simulink model "ProcessSerial"  (R2020a)
settings: Solver=FixedStepAuto  StartTime=0.0  StopTime=10.0  FixedStep=1e-3  RelTol=1e-3  EnableMultiTasking=on
libraries: frdmk64flib x5, simulink x3, etargetslib x1
settings Model: ExtModeTrigDuration=5  Creator=WinnieTrandinh  LastModifiedBy=WinnieTrandinh
settings OptimizationCC: EnhancedBackFolding=on  PassReuseOutputArgsAs=Individual arguments  ZeroExternalMemoryAtStartup=off  ZeroInternalMemoryAtStartup=off  MaxStackSize=64  OptimizeBlockOrder=speed  DifferentSizesBufferReuse=on  OptimizationCustomize=off  EfficientTunableParamExpr=on
settings DebuggingCC: ParameterTunabilityLossMsg=error
settings HardwareCC: ProdBitPerPointer=32  ProdBitPerSizeT=32  ProdBitPerPtrDiffT=32  ProdLargestAtomicInteger=Long  ProdLargestAtomicFloat=Double  ProdWordSize=32  ProdHWDeviceType=ARM Compatible->ARM Cortex
settings SFSimCC: MATLABDynamicMemAlloc=off
settings RTWCC: SystemTargetFile=ert.tlc  HardwareBoard=NXP FRDM-K64F  TemplateMakefile=ert_default_tmf  Toolchain=GNU Tools for ARM Embedded Processors
settings CodeAppCC: ForceParamTrailComments=on  IgnoreCustomStorageClasses=off  OperatorAnnotations=on  SimulinkDataObjDesc=on  SFDataObjDesc=on  InsertBlockDesc=on

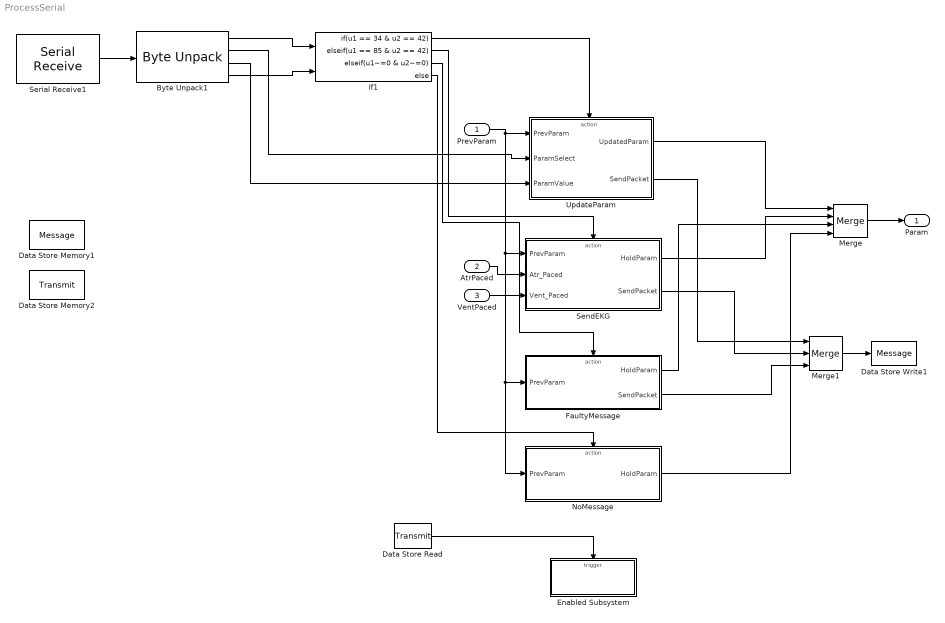
== system ProcessSerial ==
  PrevParam : Inport
  AtrPaced : Inport  Port=2
  VentPaced : Inport  Port=3
  Byte Unpack1 : etargetslib/Byte Unpack  dimensions={1 1 1 1}  datatypes={'uint8', 'uint8', 'single', 'uint8'}  byteAlign=1
  Data Store Memory1 : DataStoreMemory  DataStoreName=Message  ReadBeforeWriteMsg=warning  WriteAfterWriteMsg=warning  WriteAfterReadMsg=warning  InitialValue=[0; 0; 0; 0; 0; 0; 0; 0; 0; 0; 0; 0; 0; 0; 0; 0]  ShowAdditionalParam=off  OutDataTypeStr=uint8
  Data Store Memory2 : DataStoreMemory  DataStoreName=Transmit  ReadBeforeWriteMsg=warning  WriteAfterWriteMsg=warning  WriteAfterReadMsg=warning  ShowAdditionalParam=off
  Data Store Read : DataStoreRead  DataStoreName=Transmit
  Data Store Write1 : DataStoreWrite  DataStoreName=Message
  Enabled Subsystem : Subsystem  TreatAsAtomicUnit=on
  FaultyMessage : Subsystem  TreatAsAtomicUnit=on
  If1 : If  NumInputs=2  IfExpression=u1 == 34 & u2 == 42  ElseIfExpressions=u1 == 85 & u2 == 42, u1~=0 & u2~=0
  Merge : Merge  Inputs=4
  Merge1 : Merge  Inputs=3
  NoMessage : Subsystem  TreatAsAtomicUnit=on
  SendEKG : Subsystem  TreatAsAtomicUnit=on
  Serial Receive1 : frdmk64flib/Serial Receive  SCIModule=0  Baudrate=uint32(9600)  Parity=None  StopBits=1  HardwareFlowControl=None  ByteOrder=LittleEndian  DataType=uint8  DataLength=7  BlockingMode=off  OutputStatus=off  SampleTime=-1
  UpdateParam : Subsystem
  Param : Outport
  wires:
  Byte Unpack1/1 -> If1/1
  PrevParam/1 -> NoMessage/1(PrevParam), FaultyMessage/1(PrevParam), SendEKG/1(PrevParam), UpdateParam/1(PrevParam)
  Byte Unpack1/2 -> UpdateParam/2(ParamSelect)
  Byte Unpack1/3 -> UpdateParam/3(ParamValue)
  Byte Unpack1/4 -> If1/2
  If1/1 -> UpdateParam/Action
  Serial Receive1/1 -> Byte Unpack1/1
  Merge/1 -> Param/1
  UpdateParam/1(UpdatedParam) -> Merge/1
  If1/2 -> SendEKG/Action
  SendEKG/1(HoldParam) -> Merge/2
  VentPaced/1 -> SendEKG/3(Vent_Paced)
  AtrPaced/1 -> SendEKG/2(Atr_Paced)
  UpdateParam/2(SendPacket) -> Merge1/1
  SendEKG/2(SendPacket) -> Merge1/2
  FaultyMessage/2(SendPacket) -> Merge1/3
  Data Store Read/1 -> Enabled Subsystem/Trigger
  Merge1/1 -> Data Store Write1/1
  If1/3 -> FaultyMessage/Action
  FaultyMessage/1(HoldParam) -> Merge/3
  If1/4 -> NoMessage/Action
  NoMessage/1(HoldParam) -> Merge/4

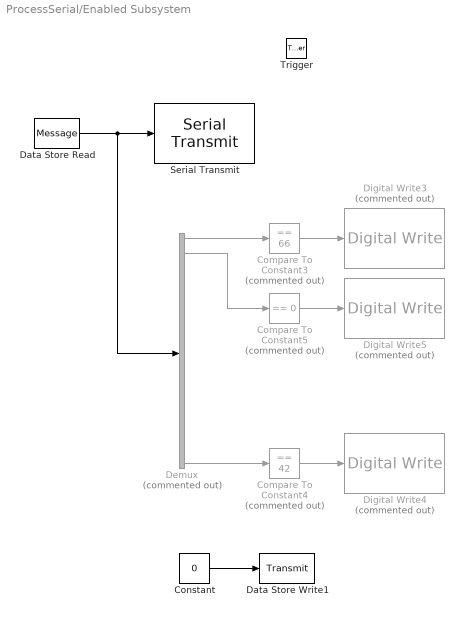
== system ProcessSerial/Enabled Subsystem ==
  Trigger : TriggerPort  VariantControl=Variant  PortDimensions=1
  Compare To Constant3 : simulink/Logic and Bit Operations/Compare To Constant  Commented=on  relop===  const=66  OutDataTypeStr=boolean
  Compare To Constant4 : simulink/Logic and Bit Operations/Compare To Constant  Commented=on  relop===  const=42  OutDataTypeStr=boolean
  Compare To Constant5 : simulink/Logic and Bit Operations/Compare To Constant  Commented=on  relop===  const=0  OutDataTypeStr=boolean
  Constant : Constant  Value=0
  Data Store Read : DataStoreRead  DataStoreName=Message
  Data Store Write1 : DataStoreWrite  DataStoreName=Transmit
  Demux : Demux  Commented=on  Outputs=16
  Digital Write3 : frdmk64flib/Digital Write  Commented=on  Whichpin=RED_LED
  Digital Write4 : frdmk64flib/Digital Write  Commented=on  Whichpin=GREEN_LED
  Digital Write5 : frdmk64flib/Digital Write  Commented=on  Whichpin=BLUE_LED
  Serial Transmit : frdmk64flib/Serial Transmit  SCIModule=0  Baudrate=uint32(9600)  Parity=None  StopBits=1  HardwareFlowControl=None  ByteOrder=LittleEndian  BlockingMode=on  OutputStatus=off
  wires:
  Compare To Constant4/1 -> Digital Write4/1
  Compare To Constant5/1 -> Digital Write5/1
  Demux/1 -> Compare To Constant3/1
  Compare To Constant3/1 -> Digital Write3/1
  Demux/16 -> Compare To Constant4/1
  Demux/2 -> Compare To Constant5/1
  Data Store Read/1 -> Demux/1, Serial Transmit/1
  Constant/1 -> Data Store Write1/1

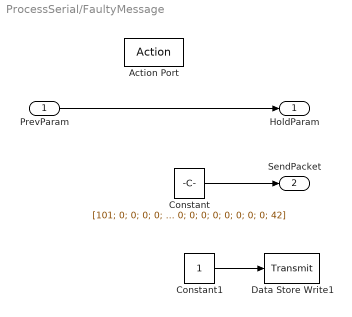
== system ProcessSerial/FaultyMessage ==
  PrevParam : Inport
  Action Port : ActionPort  ActionPortLabel=elseif( u1~=0 & u2~=0)
  Constant : Constant  Value=[101; 0; 0; 0; 0; 0; 0; 0; 0; 0; 0; 0; 0; 0; 0; 42]  OutDataTypeStr=uint8
  Constant1 : Constant
  Data Store Write1 : DataStoreWrite  DataStoreName=Transmit
  HoldParam : Outport
  SendPacket : Outport  Port=2
  wires:
  PrevParam/1 -> HoldParam/1
  Constant/1 -> SendPacket/1
  Constant1/1 -> Data Store Write1/1

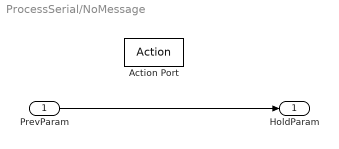
== system ProcessSerial/NoMessage ==
  PrevParam : Inport
  Action Port : ActionPort  ActionPortLabel=else
  HoldParam : Outport
  wires:
  PrevParam/1 -> HoldParam/1

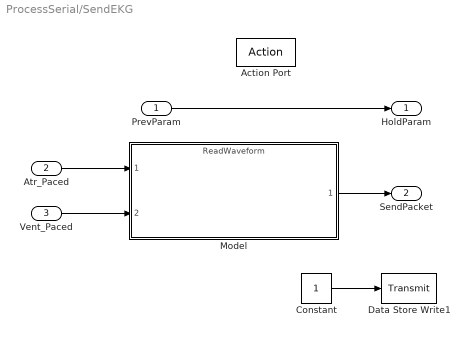
== system ProcessSerial/SendEKG ==
  PrevParam : Inport
  Atr_Paced : Inport  Port=2  OutDataTypeStr=uint8
  Vent_Paced : Inport  Port=3  OutDataTypeStr=uint8
  Action Port : ActionPort  ActionPortLabel=elseif(u1 == 85 & u2 == 42)
  Constant : Constant
  Data Store Write1 : DataStoreWrite  DataStoreName=Transmit
  Model : ModelReference  ModelNameDialog=ReadWaveform.slx  SimulationMode=Normal  ModelReferenceVersion=1.9
  HoldParam : Outport
  SendPacket : Outport  Port=2
  wires:
  PrevParam/1 -> HoldParam/1
  Model/1 -> SendPacket/1
  Atr_Paced/1 -> Model/1
  Vent_Paced/1 -> Model/2
  Constant/1 -> Data Store Write1/1

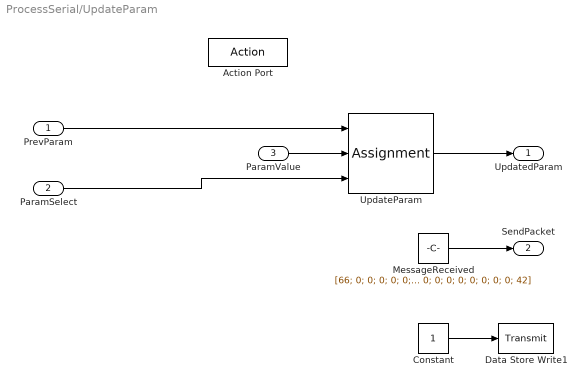
== system ProcessSerial/UpdateParam ==
  PrevParam : Inport  OutDataTypeStr=single  PortDimensions=[1 19]
  ParamSelect : Inport  Port=2
  ParamValue : Inport  Port=3
  Action Port : ActionPort  ActionPortLabel=if(u1 == 34 & u2 == 42)
  Constant : Constant
  Data Store Write1 : DataStoreWrite  DataStoreName=Transmit
  MessageReceived : Constant  Value=[66; 0; 0; 0; 0; 0; 0; 0; 0; 0; 0; 0; 0; 0; 0; 42]  OutDataTypeStr=uint8
  UpdateParam : Assignment  DiagnosticForDimensions=Warning  IndexOptions=Index vector (port)  Indices=1  OutputSizes=1
  UpdatedParam : Outport
  SendPacket : Outport  Port=2
  wires:
  PrevParam/1 -> UpdateParam/1
  UpdateParam/1 -> UpdatedParam/1
  ParamSelect/1 -> UpdateParam/3
  ParamValue/1 -> UpdateParam/2
  Constant/1 -> Data Store Write1/1
  MessageReceived/1 -> SendPacket/1
